simulink model "nid_cvst_motion"  (Simulink 10.0)
settings: Solver=FixedStepDiscrete  StartTime=0.0  StopTime=inf  RelTol=1e-3  EnableMultiTasking=on
libraries: vipsnks x2, nid_lib x2
settings Model: Creator=tchikama  LastModifiedBy=bhisma
settings DataIOCC: LimitDataPoints=on  SignalLoggingSaveFormat=ModelDataLogs  SaveOutput=off
settings OptimizationCC: ExpressionDepthLimit=2147483647  SimCompilerOptimization=on
settings DebuggingCC: SolverPrmCheckMsg=warning  FcnCallInpInsideContextMsg=warning  StateNameClashWarn=warning
settings HardwareCC: ProdIntDivRoundTo=Zero  ProdEndianess=LittleEndian  ProdHWDeviceType=Generic->32-bit x86 compatible
settings RTWCC: RTWCompilerOptimization=on
settings CodeAppCC: MaxIdLength=95
settings GRTTargetCC: GeneratePreprocessorConditionals=Disable all
settings ConfigComp: CovExternalEMLEnable=off

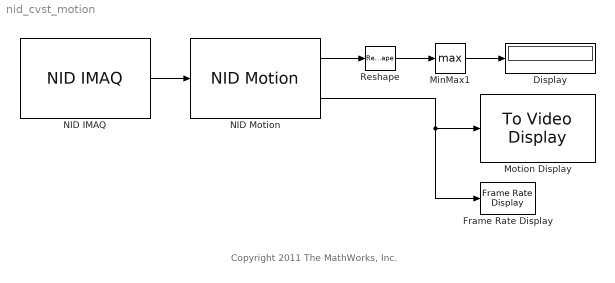
== system nid_cvst_motion ==
  note: Copyright 2011 The MathWorks, Inc.
  Display : Display
  Frame Rate Display : vipsnks/Frame Rate Display  UpdateRate=10
      settings: SourceProductName=Computer Vision Toolbox  SourceProductBaseCode=VP
  MinMax1 : MinMax  Function=max
  Motion Display : vipsnks/To Video Display  inputType=Obsolete  imagePorts=One multidimensional signal  OutputDevice=On-screen video monitor  fullScreen=off  videoWindowX=856  videoWindowY=113  saveWindowSize=off  videoWindowWidth=640  videoWindowHeight=480  dataOrg=Column-major  openAtMdlStart=on  isWindowOpen=on
      settings: SourceProductName=Computer Vision Toolbox  SourceProductBaseCode=VP
  NID IMAQ : nid_lib/NID IMAQ  imaq_depth=off  imaq_motion=on  imaq_image=off  view_point=off  imaq_skeleton=off  imaq_ir=off  mirror_image=off  imaq_sample_time=1/30  res_fps=VGA (640x480): 30 FPS  angle=0  angle_read=off  near_mode=off
  NID Motion : nid_lib/NID Motion  viewer=on
  Reshape : Reshape
  wires:
  NID IMAQ/1 -> NID Motion/1
  NID Motion/1 -> Reshape/1
  Reshape/1 -> MinMax1/1
  MinMax1/1 -> Display/1
  NID Motion/2 -> Frame Rate Display/1, Motion Display/1
